simulink model "accurate_sim"  (R2020b)
settings: Solver=VariableStepAuto  StartTime=0.0  StopTime=10.0  RelTol=1e-3
undefined symbols (not defined in the file): const, mech, pid
settings Model: Creator=Utente  LastModifiedBy=Utente

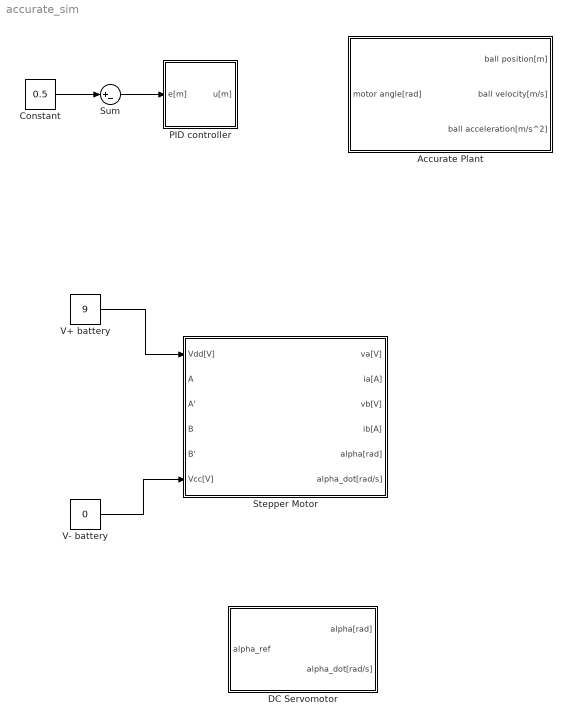
== system accurate_sim ==
  Accurate Plant : Subsystem
  Constant : Constant  Value=0.5
  DC Servomotor : Subsystem
  "PID controller " : Subsystem
  Stepper Motor : Subsystem
  Sum : Sum  Inputs=|+-
  V+ battery : Constant  Value=9
  V- battery : Constant  Value=0
  wires:
  Sum/1 -> "PID controller "/1(e[m])
  Constant/1 -> Sum/1
  V- battery/1 -> Stepper Motor/6(Vcc[V])
  V+ battery/1 -> Stepper Motor/1(Vdd[V])

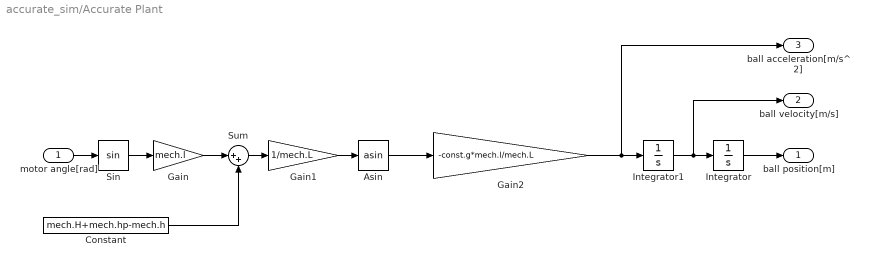
== system accurate_sim/Accurate Plant ==
  motor angle[rad] : Inport
  Asin : Trigonometry  Operator=asin
  Constant : Constant  Value=mech.H+mech.hp-mech.h
  Gain : Gain  Gain=mech.l
  Gain1 : Gain  Gain=1/mech.L
  Gain2 : Gain  Gain=-const.g*mech.l/mech.L
  Integrator : Integrator
  Integrator1 : Integrator
  Sin : Trigonometry
  Sum : Sum  Inputs=|++
  ball position[m] : Outport
  ball velocity[m/s] : Outport  Port=2
  ball acceleration[m/s^2] : Outport  Port=3
  wires:
  Integrator/1 -> ball position[m]/1
  Integrator1/1 -> ball velocity[m/s]/1, Integrator/1
  Gain2/1 -> ball acceleration[m/s^2]/1, Integrator1/1
  motor angle[rad]/1 -> Sin/1
  Sin/1 -> Gain/1
  Gain/1 -> Sum/1
  Constant/1 -> Sum/2
  Gain1/1 -> Asin/1
  Sum/1 -> Gain1/1
  Asin/1 -> Gain2/1

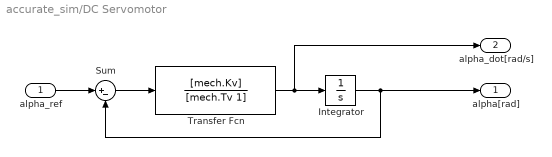
== system accurate_sim/DC Servomotor ==
  alpha_ref : Inport
  Integrator : Integrator
  Sum : Sum  Inputs=|+-
  Transfer Fcn : TransferFcn  Numerator=[mech.Kv]  Denominator=[mech.Tv 1]
  alpha[rad] : Outport
  alpha_dot[rad/s] : Outport  Port=2
  wires:
  Integrator/1 -> Sum/2, alpha[rad]/1
  alpha_ref/1 -> Sum/1
  Sum/1 -> Transfer Fcn/1
  Transfer Fcn/1 -> Integrator/1, alpha_dot[rad/s]/1

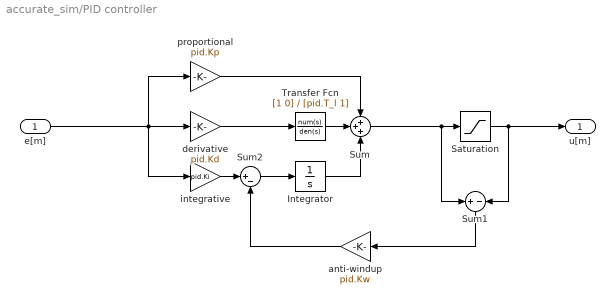
== system accurate_sim/PID controller  ==
  e[m] : Inport  Unit=deg
  Integrator : Integrator
  Saturation : Saturate  UpperLimit=30  LowerLimit=-30
  Sum : Sum  Inputs=+++
  Sum1 : Sum  Inputs=+|-
  Sum2 : Sum  Inputs=|+-
  Transfer Fcn : TransferFcn  Numerator=[1 0]  Denominator=[pid.T_l 1]
  anti-windup : Gain  Gain=pid.Kw
  derivative : Gain  Gain=pid.Kd
  integrative : Gain  Gain=pid.Ki
  proportional : Gain  Gain=pid.Kp
  u[m] : Outport
  wires:
  e[m]/1 -> integrative/1, derivative/1, proportional/1
  proportional/1 -> Sum/1
  Saturation/1 -> u[m]/1, Sum1/2
  integrative/1 -> Sum2/1
  Sum2/1 -> Integrator/1
  anti-windup/1 -> Sum2/2
  Integrator/1 -> Sum/3
  Transfer Fcn/1 -> Sum/2
  derivative/1 -> Transfer Fcn/1
  Sum1/1 -> anti-windup/1
  Sum/1 -> Saturation/1, Sum1/1

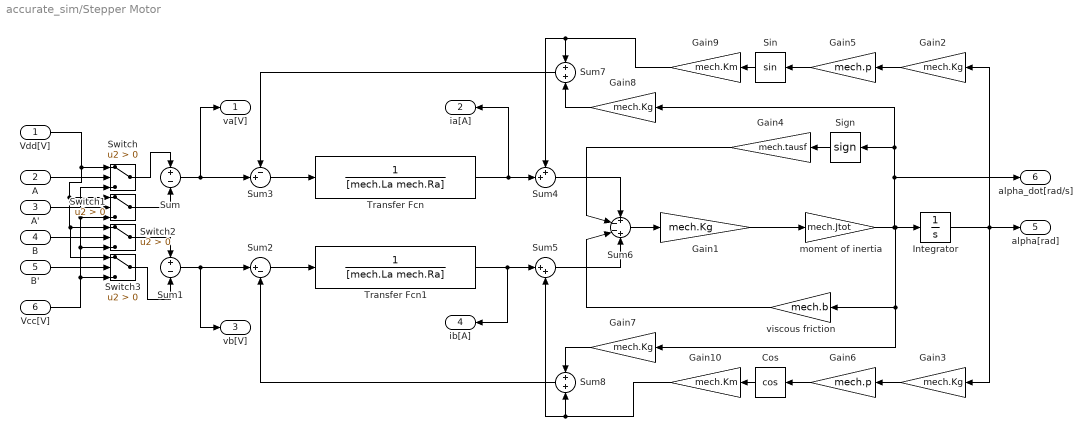
== system accurate_sim/Stepper Motor ==
  Vdd[V] : Inport
  A : Inport  Port=2
  A' : Inport  Port=3
  B : Inport  Port=4
  B' : Inport  Port=5
  Vcc[V] : Inport  Port=6
  Cos : Trigonometry  Operator=cos
  Gain{1..3,7..8} (5 alike) : Gain  Gain=mech.Kg
  Gain10 : Gain  Gain=mech.Km
  Gain4 : Gain  Gain=mech.tausf
  Gain5 : Gain  Gain=mech.p
  Gain6 : Gain  Gain=mech.p
  Gain9 : Gain  Gain=mech.Km
  Integrator : Integrator
  Sign : Signum
  Sin : Trigonometry
  Sum : Sum  Inputs=+|-
  Sum1 : Sum  Inputs=+|-
  Sum2 : Sum  Inputs=|+-
  Sum3 : Sum  Inputs=-+|
  Sum4 : Sum  Inputs=++|
  Sum5 : Sum  Inputs=|++
  Sum6 : Sum  Inputs=+--+
  Sum7 : Sum
  Sum8 : Sum
  Switch{,1..3} (4 alike) : Switch  Criteria=u2 > Threshold
  Transfer Fcn : TransferFcn  Denominator=[mech.La mech.Ra]
  Transfer Fcn1 : TransferFcn  Denominator=[mech.La mech.Ra]
  moment of inertia : Gain  Gain=mech.Jtot
  viscous friction : Gain  Gain=mech.b
  va[V] : Outport
  ia[A] : Outport  Port=2
  vb[V] : Outport  Port=3
  ib[A] : Outport  Port=4
  alpha[rad] : Outport  Port=5
  alpha_dot[rad/s] : Outport  Port=6
  wires:
  A/1 -> Switch/2
  Vdd[V]/1 -> Switch3/1, Switch2/1, Switch1/1, Switch/1
  Vcc[V]/1 -> Switch3/3, Switch2/3, Switch1/3, Switch/3
  A'/1 -> Switch1/2
  B/1 -> Switch2/2
  B'/1 -> Switch3/2
  Switch1/1 -> Sum/2
  Switch/1 -> Sum/1
  Sum/1 -> Sum3/2, va[V]/1
  Switch2/1 -> Sum1/1
  Switch3/1 -> Sum1/2
  Sum1/1 -> Sum2/1, vb[V]/1
  Integrator/1 -> Gain3/1, Gain2/1, alpha[rad]/1
  Sum3/1 -> Transfer Fcn/1
  Sum2/1 -> Transfer Fcn1/1
  Sum4/1 -> Sum6/1
  Sum5/1 -> Sum6/4
  Sum6/1 -> Gain1/1
  Gain1/1 -> moment of inertia/1
  moment of inertia/1 -> viscous friction/1, Gain7/1, Integrator/1, Sign/1, Gain8/1, alpha_dot[rad/s]/1
  viscous friction/1 -> Sum6/3
  Gain4/1 -> Sum6/2
  Transfer Fcn/1 -> ia[A]/1, Sum4/2
  Transfer Fcn1/1 -> ib[A]/1, Sum5/1
  Gain2/1 -> Gain5/1
  Gain5/1 -> Sin/1
  Gain6/1 -> Cos/1
  Gain3/1 -> Gain6/1
  Gain8/1 -> Sum7/2
  Sin/1 -> Gain9/1
  Gain7/1 -> Sum8/1
  Cos/1 -> Gain10/1
  Sum8/1 -> Sum2/2
  Sum7/1 -> Sum3/1
  Gain9/1 -> Sum4/1, Sum7/1
  Gain10/1 -> Sum8/2, Sum5/2
  Sign/1 -> Gain4/1
